simulink model "MEMS_Gyro_Structure_Model_231114"  (R2022b)
settings: Solver=VariableStepAuto  StartTime=0.0  StopTime=3  MaxStep=1e-5  RelTol=1e-3
libraries: cstblocks x1
settings Model: Creator=admin  LastModifiedBy=Rio

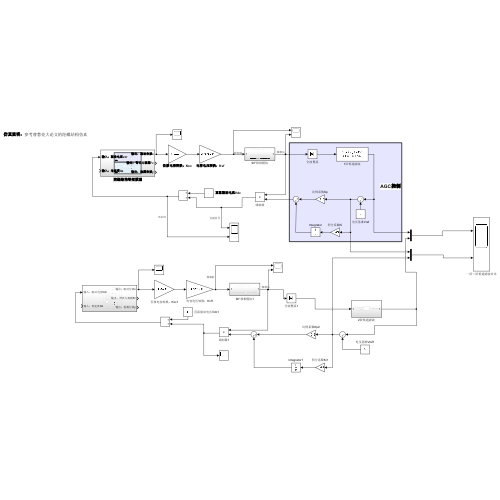
[thumbnail: Simulink's stored preview of the top-level diagram]
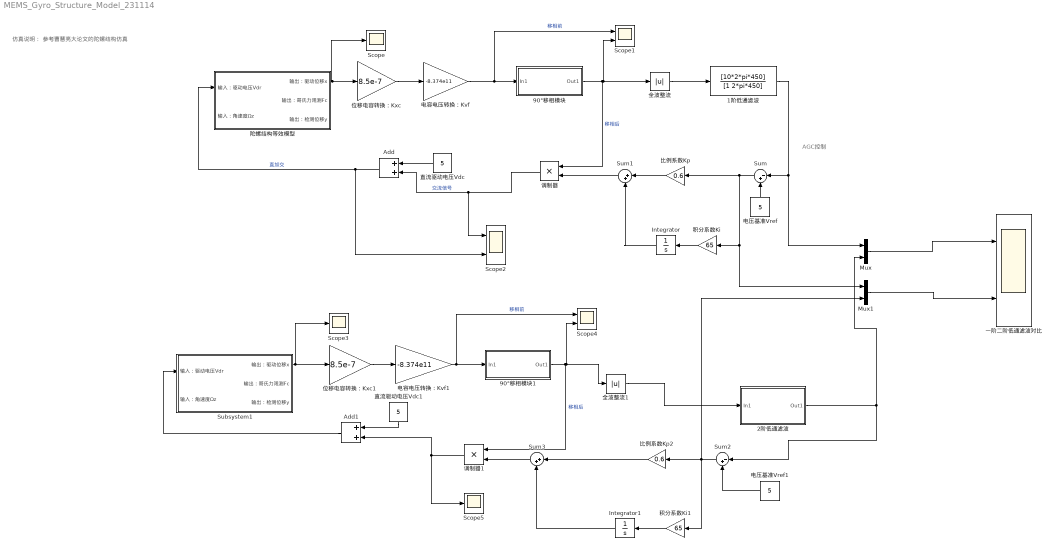
== system MEMS_Gyro_Structure_Model_231114 ==
  note: 仿真说明： 参考曹慧亮大论文的陀螺结构仿真
  note: AGC控制
  1阶低通滤波 : TransferFcn  Numerator=[10*2*pi*450]  Denominator=[1 2*pi*450]
  2阶低通滤波 : Subsystem
  90°移相模块 : Subsystem
  90°移相模块1 : Subsystem
  Add : Sum
  Add1 : Sum
  Integrator : Integrator
  Integrator1 : Integrator
  Mux : Mux  Inputs=2
  Mux1 : Mux  Inputs=2
  Scope : Scope
  Scope1 : Scope  NumInputPorts=2
  Scope2 : Scope  NumInputPorts=2
  Scope3 : Scope
  Scope4 : Scope  NumInputPorts=2
  Scope5 : Scope
  Subsystem1 : Subsystem
  Sum : Sum  Inputs=|-+
  Sum1 : Sum  Inputs=|++
  Sum2 : Sum  Inputs=|-+
  Sum3 : Sum  Inputs=|++
  一阶二阶低通滤波对比 : Scope  NumInputPorts=2
  位移电容转换：Kxc : Gain  Gain=8.5e-7
  位移电容转换：Kxc1 : Gain  Gain=8.5e-7
  全波整流 : Abs  SaturateOnIntegerOverflow=off
  全波整流1 : Abs  SaturateOnIntegerOverflow=off
  比例系数Kp : Gain  Gain=0.6
  比例系数Kp2 : Gain  Gain=0.6
  电压基准Vref : Constant  Value=5
  电压基准Vref1 : Constant  Value=5
  电容电压转换：Kvf : Gain  Gain=-8.374e11
  电容电压转换：Kvf1 : Gain  Gain=-8.374e11
  直流驱动电压Vdc : Constant  Value=5
  直流驱动电压Vdc1 : Constant  Value=5
  积分系数Ki : Gain  Gain=65
  积分系数Ki1 : Gain  Gain=65
  调制器 : Product
  调制器1 : Product
  陀螺结构等效模型 : Subsystem
  wires:
  Add/1 -> 陀螺结构等效模型/1(输入：驱动电压Vdr), Scope2/2  "直加交"
  陀螺结构等效模型/1(输出：驱动位移x) -> Scope/1, 位移电容转换：Kxc/1
  90°移相模块/1(Out1) -> 全波整流/1, Scope1/2, 调制器/1  "移相后"
  位移电容转换：Kxc/1 -> 电容电压转换：Kvf/1
  电容电压转换：Kvf/1 -> Scope1/1, 90°移相模块/1(In1)  "移相前"
  Sum1/1 -> 调制器/2
  直流驱动电压Vdc/1 -> Add/1
  调制器/1 -> Scope2/1, Add/2  "交流信号"
  全波整流/1 -> 1阶低通滤波/1
  比例系数Kp/1 -> Sum1/1
  电压基准Vref/1 -> Sum/2
  Sum/1 -> 比例系数Kp/1, Mux1/1, 积分系数Ki/1
  Integrator/1 -> Sum1/2
  积分系数Ki/1 -> Integrator/1
  1阶低通滤波/1 -> Mux/1, Sum/1
  积分系数Ki1/1 -> Integrator1/1
  Integrator1/1 -> Sum3/2
  Sum2/1 -> Mux1/2, 积分系数Ki1/1, 比例系数Kp2/1
  电压基准Vref1/1 -> Sum2/2
  比例系数Kp2/1 -> Sum3/1
  调制器1/1 -> Scope5/1, Add1/2
  直流驱动电压Vdc1/1 -> Add1/1
  Sum3/1 -> 调制器1/2
  电容电压转换：Kvf1/1 -> 90°移相模块1/1(In1), Scope4/1  "移相前"
  位移电容转换：Kxc1/1 -> 电容电压转换：Kvf1/1
  90°移相模块1/1(Out1) -> 调制器1/1, Scope4/2, 全波整流1/1  "移相后"
  Subsystem1/1(输出：驱动位移x) -> 位移电容转换：Kxc1/1, Scope3/1
  Add1/1 -> Subsystem1/1(输入：驱动电压Vdr)
  Mux/1 -> 一阶二阶低通滤波对比/1
  Mux1/1 -> 一阶二阶低通滤波对比/2
  2阶低通滤波/1(Out1) -> Mux/2, Sum2/1
  全波整流1/1 -> 2阶低通滤波/1(In1)

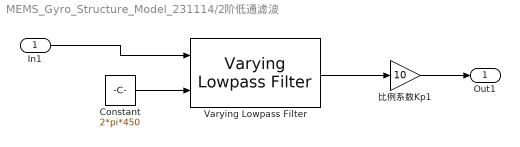
== system MEMS_Gyro_Structure_Model_231114/2阶低通滤波 ==
  In1 : Inport
  Constant : Constant  Value=2*pi*450
  Varying Lowpass Filter : cstblocks/Linear Parameter Varying/Varying Lowpass Filter  N=2
  比例系数Kp1 : Gain  Gain=10
  Out1 : Outport
  wires:
  Constant/1 -> Varying Lowpass Filter/2
  Varying Lowpass Filter/1 -> 比例系数Kp1/1
  比例系数Kp1/1 -> Out1/1
  In1/1 -> Varying Lowpass Filter/1

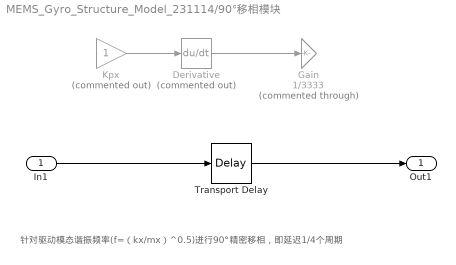
== system MEMS_Gyro_Structure_Model_231114/90°移相模块 ==
  note: 针对驱动模态谐振频率(f=（kx/mx）^0.5)进行90°精密移相，即延迟1/4个周期
  In1 : Inport
  Derivative : Derivative  Commented=on
  Gain : Gain  Commented=through  Gain=1/3333
  Kpx : Gain  Commented=on
  Transport Delay : TransportDelay  DelayTime=1/(3489.44*4)
  Out1 : Outport
  wires:
  In1/1 -> Transport Delay/1
  Transport Delay/1 -> Out1/1
  Derivative/1 -> Gain/1
  Kpx/1 -> Derivative/1

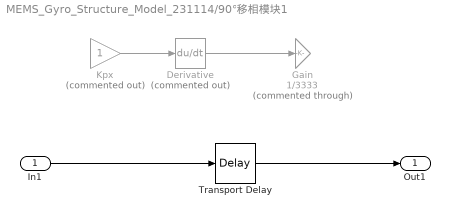
== system MEMS_Gyro_Structure_Model_231114/90°移相模块1 ==
  In1 : Inport
  Derivative : Derivative  Commented=on
  Gain : Gain  Commented=through  Gain=1/3333
  Kpx : Gain  Commented=on
  Transport Delay : TransportDelay  DelayTime=1/(3489.44*4)
  Out1 : Outport
  wires:
  Kpx/1 -> Derivative/1
  Derivative/1 -> Gain/1
  Transport Delay/1 -> Out1/1
  In1/1 -> Transport Delay/1

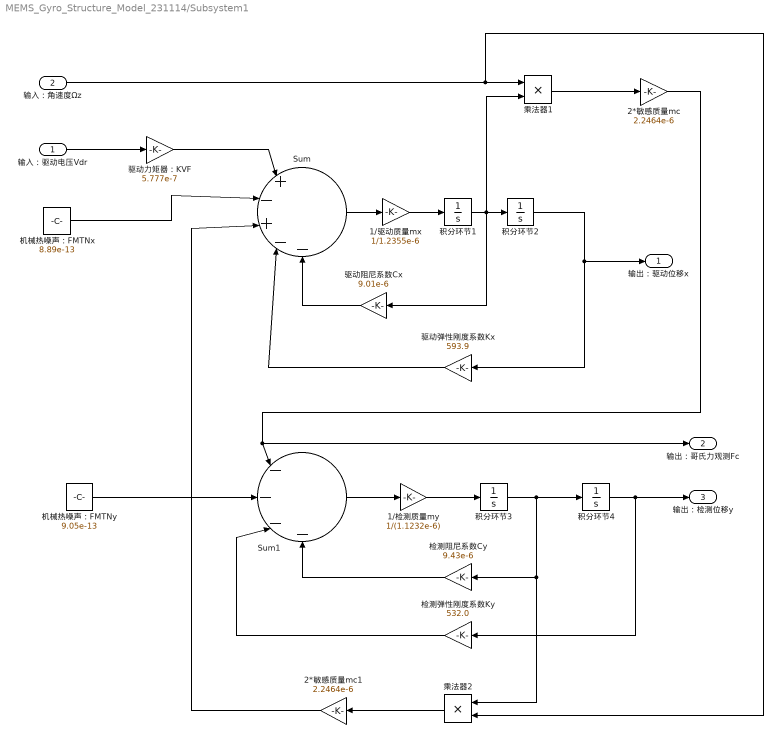
== system MEMS_Gyro_Structure_Model_231114/Subsystem1 ==
  输入：驱动电压Vdr : Inport
  输入：角速度Ωz : Inport  Port=2
  1/检测质量my : Gain  Gain=1/(1.1232e-6)
  1/驱动质量mx : Gain  Gain=1/1.2355e-6
  2*敏感质量mc : Gain  Gain=2.2464e-6
  2*敏感质量mc1 : Gain  Gain=2.2464e-6
  Sum : Sum  Inputs=|+-+--
  Sum1 : Sum  Inputs=|----
  乘法器1 : Product
  乘法器2 : Product
  机械热噪声：FMTNx : Constant  Value=8.89e-13
  机械热噪声：FMTNy : Constant  Value=9.05e-13
  检测弹性刚度系数Ky : Gain  Gain=532.0
  检测阻尼系数Cy : Gain  Gain=9.43e-6
  积分环节{1..4} (4 alike) : Integrator
  驱动力矩器：KVF : Gain  Gain=5.777e-7
  驱动弹性刚度系数Kx : Gain  Gain=593.9
  驱动阻尼系数Cx : Gain  Gain=9.01e-6
  输出：驱动位移x : Outport
  输出：哥氏力观测Fc : Outport  Port=2
  输出：检测位移y : Outport  Port=3
  wires:
  检测阻尼系数Cy/1 -> Sum1/4
  乘法器2/1 -> 2*敏感质量mc1/1
  1/驱动质量mx/1 -> 积分环节1/1
  驱动力矩器：KVF/1 -> Sum/1
  乘法器1/1 -> 2*敏感质量mc/1
  驱动弹性刚度系数Kx/1 -> Sum/4
  2*敏感质量mc1/1 -> Sum/3
  驱动阻尼系数Cx/1 -> Sum/5
  Sum/1 -> 1/驱动质量mx/1
  输入：角速度Ωz/1 -> 乘法器1/1, 乘法器2/2
  积分环节2/1 -> 驱动弹性刚度系数Kx/1, 输出：驱动位移x/1
  机械热噪声：FMTNy/1 -> Sum1/2
  输入：驱动电压Vdr/1 -> 驱动力矩器：KVF/1
  Sum1/1 -> 1/检测质量my/1
  检测弹性刚度系数Ky/1 -> Sum1/3
  积分环节3/1 -> 积分环节4/1, 检测阻尼系数Cy/1, 乘法器2/1
  2*敏感质量mc/1 -> Sum1/1, 输出：哥氏力观测Fc/1
  机械热噪声：FMTNx/1 -> Sum/2
  积分环节4/1 -> 检测弹性刚度系数Ky/1, 输出：检测位移y/1
  积分环节1/1 -> 积分环节2/1, 乘法器1/2, 驱动阻尼系数Cx/1
  1/检测质量my/1 -> 积分环节3/1

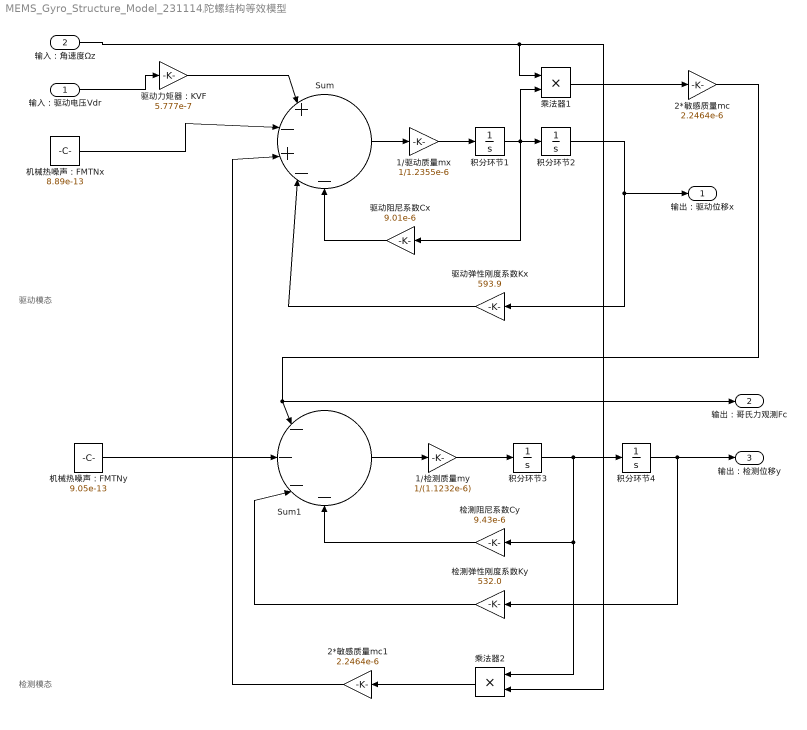
== system MEMS_Gyro_Structure_Model_231114/陀螺结构等效模型 ==
  note: 检测模态
  note: 驱动模态
  输入：驱动电压Vdr : Inport
  输入：角速度Ωz : Inport  Port=2
  1/检测质量my : Gain  Gain=1/(1.1232e-6)
  1/驱动质量mx : Gain  Gain=1/1.2355e-6
  2*敏感质量mc : Gain  Gain=2.2464e-6
  2*敏感质量mc1 : Gain  Gain=2.2464e-6
  Sum : Sum  Inputs=|+-+--
  Sum1 : Sum  Inputs=|----
  乘法器1 : Product
  乘法器2 : Product
  机械热噪声：FMTNx : Constant  Value=8.89e-13
  机械热噪声：FMTNy : Constant  Value=9.05e-13
  检测弹性刚度系数Ky : Gain  Gain=532.0
  检测阻尼系数Cy : Gain  Gain=9.43e-6
  积分环节{1..4} (4 alike) : Integrator
  驱动力矩器：KVF : Gain  Gain=5.777e-7
  驱动弹性刚度系数Kx : Gain  Gain=593.9
  驱动阻尼系数Cx : Gain  Gain=9.01e-6
  输出：驱动位移x : Outport
  输出：哥氏力观测Fc : Outport  Port=2
  输出：检测位移y : Outport  Port=3
  wires:
  1/检测质量my/1 -> 积分环节3/1
  积分环节1/1 -> 驱动阻尼系数Cx/1, 乘法器1/2, 积分环节2/1
  积分环节4/1 -> 输出：检测位移y/1, 检测弹性刚度系数Ky/1
  机械热噪声：FMTNx/1 -> Sum/2
  2*敏感质量mc/1 -> 输出：哥氏力观测Fc/1, Sum1/1
  积分环节3/1 -> 乘法器2/1, 检测阻尼系数Cy/1, 积分环节4/1
  检测弹性刚度系数Ky/1 -> Sum1/3
  Sum1/1 -> 1/检测质量my/1
  输入：驱动电压Vdr/1 -> 驱动力矩器：KVF/1
  机械热噪声：FMTNy/1 -> Sum1/2
  积分环节2/1 -> 输出：驱动位移x/1, 驱动弹性刚度系数Kx/1
  输入：角速度Ωz/1 -> 乘法器2/2, 乘法器1/1
  Sum/1 -> 1/驱动质量mx/1
  驱动阻尼系数Cx/1 -> Sum/5
  2*敏感质量mc1/1 -> Sum/3
  驱动弹性刚度系数Kx/1 -> Sum/4
  乘法器1/1 -> 2*敏感质量mc/1
  驱动力矩器：KVF/1 -> Sum/1
  1/驱动质量mx/1 -> 积分环节1/1
  乘法器2/1 -> 2*敏感质量mc1/1
  检测阻尼系数Cy/1 -> Sum1/4
